simulink model "testHoldUntil"  (R2014a)
settings: Solver=FixedStepDiscrete  StartTime=0.0  StopTime=Inf  FixedStep=0.001  RelTol=1e-3
libraries: libButtons x2, dspswit3 x1
settings Model: BufferReuse=off  Creator=djoshea  LastModifiedBy=djoshea
settings SolverCC: EnableConcurrentExecution=on
settings OptimizationCC: BlockReduction=off  OptimizeBlockIOStorage=off  BufferReuse=off  GlobalBufferReuse=off  ExpressionFolding=off  LocalBlockOutputs=off
settings HardwareCC: ProdIntDivRoundTo=Zero  ProdEndianess=LittleEndian  ProdHWDeviceType=Generic->32-bit x86 compatible
settings RTWCC: SystemTargetFile=slrt.tlc  TemplateMakefile=slrt_default_tmf  Description=Simulink Real-Time  ProcessScript=slrt_make_rtw_hook  RTWCompilerOptimization=On
settings SimulinkRealTimeCC: GeneratePreprocessorConditionals=Disable all  EnableShiftOperators=on

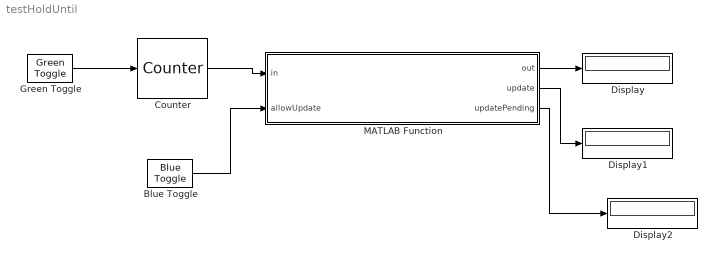
== system testHoldUntil ==
  Blue Toggle : libButtons/Blue Toggle  SystemSampleTime=-1
  Counter : dspswit3/Counter  Direction=Up  CountEvent=Non-zero sample  CounterSize=32 bits  MaxCount=255  InitialCount=0  Output=Count  HitValue=32  ResetInput=off  SamplesPerFrame=1  Ts=1  CntDtype=uint32  HitDtype=Logical
  Display : Display
  Display1 : Display
  Display2 : Display
  Green Toggle : libButtons/Green Toggle  SystemSampleTime=-1
  MATLAB Function : MATLAB Function  TreatAsAtomicUnit=on
  wires:
  Counter/1 -> MATLAB Function/1(in)
  Green Toggle/1 -> Counter/1
  Blue Toggle/1 -> MATLAB Function/2(allowUpdate)
  MATLAB Function/1(out) -> Display/1
  MATLAB Function/2(update) -> Display1/1
  MATLAB Function/3(updatePending) -> Display2/1

== matlab function testHoldUntil/MATLAB Function ==
  data: in input; out output; allowUpdate input uint8 size=1; update output uint8 size=1; updatePending output uint8 size=1
function [out, update, updatePending] = holdUntil(in, allowUpdate)
%#codegen

persistent pOut;
if isempty(pOut)
    pOut = in;
end

if ~isequal(pOut, in)
    if allowUpdate 
        pOut = in;
        update = uint8(1);
        updatePending = uint8(0);
    else
        update = uint8(0);
        updatePending = uint8(1);
    end
else
    update = uint8(0);
    updatePending = uint8(0);
end

out = pOut;
